simulink model "Task_1D"  (R2022a)
settings: Solver=VariableStepAuto  StartTime=0.0  StopTime=10.0  RelTol=1e-3
values from neighbouring files (symbols this model uses):
  L_wheel = R_robot * sin(theta_wheels)    [Parameter_Setup.m]
  R_wheel = D_wheel/2    (= 0.05)    [Parameter_Setup.m]
settings Model: Creator=jpcas  LastModifiedBy=jpcas

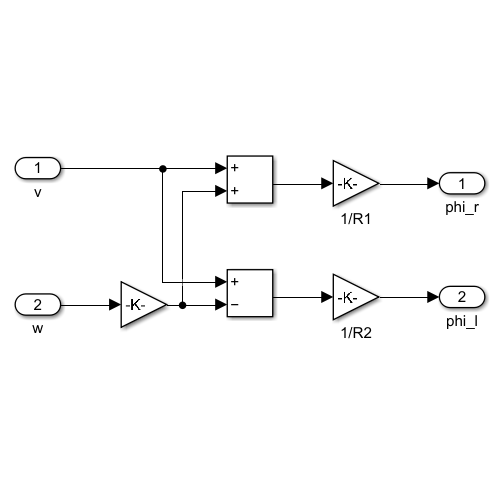
[thumbnail: Simulink's stored preview of the top-level diagram]
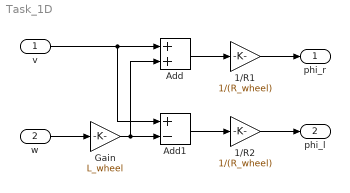
== system Task_1D ==
  v : Inport
  w : Inport  Port=2
  1/R1 : Gain  Gain=1/(R_wheel)
  1/R2 : Gain  Gain=1/(R_wheel)
  Add : Sum
  Add1 : Sum  Inputs=+-
  Gain : Gain  Gain=L_wheel
  phi_r : Outport
  phi_l : Outport  Port=2
  wires:
  v/1 -> Add1/1, Add/1
  Gain/1 -> Add/2, Add1/2
  w/1 -> Gain/1
  Add1/1 -> 1/R2/1
  Add/1 -> 1/R1/1
  1/R2/1 -> phi_l/1
  1/R1/1 -> phi_r/1
